simulink model "firefliesDemo"  (Simulink 7.4)
settings: Solver=ode3  StartTime=0.0  StopTime=200.0  FixedStep=0.5  RelTol=1e-3
values from neighbouring files (symbols this model uses):
  K = 0.1    [firefliesDemo.mat]
  N = 20    [firefliesDemo.mat]
  omega = 0.5    [firefliesDemo.mat]
  rho0 = 10    [firefliesDemo.mat]
  threshold = 4.71238898038    [firefliesDemo.mat]
  var = 10    [firefliesDemo.mat]
(part 1 of 2)
settings Model: Creator=chepeadan  LastModifiedBy=chepeadan
settings DataIOCC: SaveOutput=off  SaveState=on

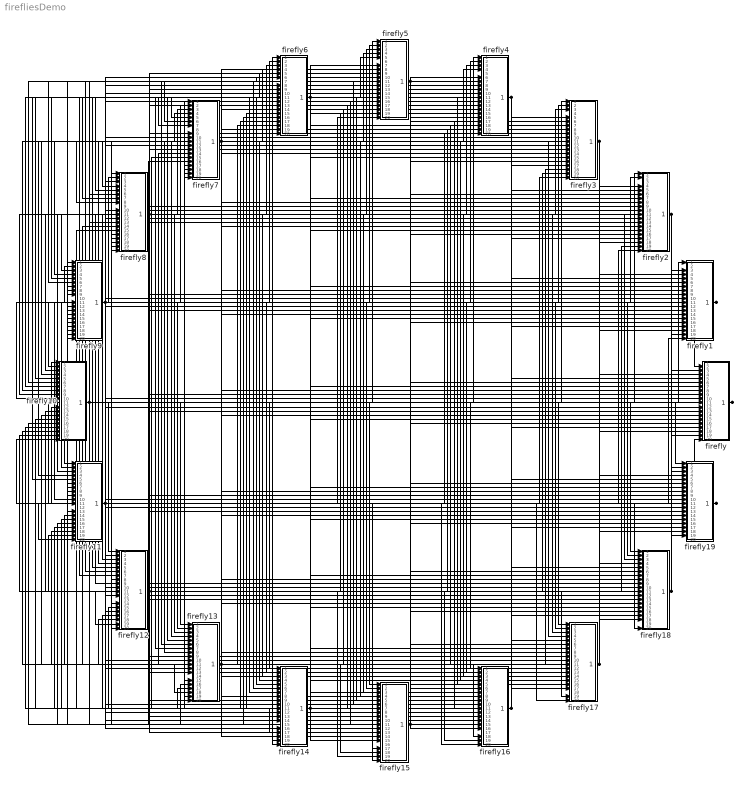
== system firefliesDemo ==
  firefly : Subsystem
  firefly1 : Subsystem
  firefly10 : Subsystem
  firefly11 : Subsystem
  firefly12 : Subsystem
  firefly13 : Subsystem
  firefly14 : Subsystem
  firefly15 : Subsystem
  firefly16 : Subsystem
  firefly17 : Subsystem
  firefly18 : Subsystem
  firefly19 : Subsystem
  firefly2 : Subsystem
  firefly3 : Subsystem
  firefly4 : Subsystem
  firefly5 : Subsystem
  firefly6 : Subsystem
  firefly7 : Subsystem
  firefly8 : Subsystem
  firefly9 : Subsystem
  wires:
  firefly/1(Out1) -> firefly1/1(In1), firefly2/1(In1), firefly3/1(In1), firefly4/1(In1), firefly5/1(In1), firefly6/1(In1), firefly7/1(In1), firefly8/1(In1), firefly9/1(In1), firefly10/1(In1), firefly11/1(In1), firefly12/1(In1), firefly13/1(In1), firefly14/1(In1), firefly15/1(In1), firefly16/1(In1), firefly17/1(In1), firefly18/1(In1), firefly19/1(In1)
  firefly1/1(Out1) -> firefly/2(In2), firefly2/2(In2), firefly3/2(In2), firefly4/2(In2), firefly5/2(In2), firefly6/2(In2), firefly7/2(In2), firefly8/2(In2), firefly9/2(In2), firefly10/2(In2), firefly11/2(In2), firefly12/2(In2), firefly13/2(In2), firefly14/2(In2), firefly15/2(In2), firefly16/2(In2), firefly17/2(In2), firefly18/2(In2), firefly19/2(In2)
  firefly2/1(Out1) -> firefly/3(In3), firefly1/3(In3), firefly3/3(In3), firefly4/3(In3), firefly5/3(In3), firefly6/3(In3), firefly7/3(In3), firefly8/3(In3), firefly9/3(In3), firefly10/3(In3), firefly11/3(In3), firefly12/3(In3), firefly13/3(In3), firefly14/3(In3), firefly15/3(In3), firefly16/3(In3), firefly17/3(In3), firefly18/3(In3), firefly19/3(In3)
  firefly3/1(Out1) -> firefly/4(In4), firefly1/4(In4), firefly2/4(In4), firefly4/4(In4), firefly5/4(In4), firefly6/4(In4), firefly7/4(In4), firefly8/4(In4), firefly9/4(In4), firefly10/4(In4), firefly11/4(In4), firefly12/4(In4), firefly13/4(In4), firefly14/4(In4), firefly15/4(In4), firefly16/4(In4), firefly17/4(In4), firefly18/4(In4), firefly19/4(In4)
  firefly4/1(Out1) -> firefly/5(In5), firefly1/5(In5), firefly2/5(In5), firefly3/5(In5), firefly5/5(In5), firefly6/5(In5), firefly7/5(In5), firefly8/5(In5), firefly9/5(In5), firefly10/5(In5), firefly11/5(In5), firefly12/5(In5), firefly13/5(In5), firefly14/5(In5), firefly15/5(In5), firefly16/5(In5), firefly17/5(In5), firefly18/5(In5), firefly19/5(In5)
  firefly5/1(Out1) -> firefly/6(In6), firefly1/6(In6), firefly2/6(In6), firefly3/6(In6), firefly4/6(In6), firefly6/6(In6), firefly7/6(In6), firefly8/6(In6), firefly9/6(In6), firefly10/6(In6), firefly11/6(In6), firefly12/6(In6), firefly13/6(In6), firefly14/6(In6), firefly15/6(In6), firefly16/6(In6), firefly17/6(In6), firefly18/6(In6), firefly19/6(In6)
  firefly6/1(Out1) -> firefly/7(In7), firefly1/7(In7), firefly2/7(In7), firefly3/7(In7), firefly4/7(In7), firefly5/7(In7), firefly7/7(In7), firefly8/7(In7), firefly9/7(In7), firefly10/7(In7), firefly11/7(In7), firefly12/7(In7), firefly13/7(In7), firefly14/7(In7), firefly15/7(In7), firefly16/7(In7), firefly17/7(In7), firefly18/7(In7), firefly19/7(In7)
  firefly7/1(Out1) -> firefly/8(In8), firefly1/8(In8), firefly2/8(In8), firefly3/8(In8), firefly4/8(In8), firefly5/8(In8), firefly6/8(In8), firefly8/8(In8), firefly9/8(In8), firefly10/8(In8), firefly11/8(In8), firefly12/8(In8), firefly13/8(In8), firefly14/8(In8), firefly15/8(In8), firefly16/8(In8), firefly17/8(In8), firefly18/8(In8), firefly19/8(In8)
  firefly8/1(Out1) -> firefly/9(In9), firefly1/9(In9), firefly2/9(In9), firefly3/9(In9), firefly4/9(In9), firefly5/9(In9), firefly6/9(In9), firefly7/9(In9), firefly9/9(In9), firefly10/9(In9), firefly11/9(In9), firefly12/9(In9), firefly13/9(In9), firefly14/9(In9), firefly15/9(In9), firefly16/9(In9), firefly17/9(In9), firefly18/9(In9), firefly19/9(In9)
  firefly9/1(Out1) -> firefly/10(In10), firefly1/10(In10), firefly2/10(In10), firefly3/10(In10), firefly4/10(In10), firefly5/10(In10), firefly6/10(In10), firefly7/10(In10), firefly8/10(In10), firefly10/10(In10), firefly11/10(In10), firefly12/10(In10), firefly13/10(In10), firefly14/10(In10), firefly15/10(In10), firefly16/10(In10), firefly17/10(In10), firefly18/10(In10), firefly19/10(In10)
  firefly10/1(Out1) -> firefly/11(In11), firefly1/11(In11), firefly2/11(In11), firefly3/11(In11), firefly4/11(In11), firefly5/11(In11), firefly6/11(In11), firefly7/11(In11), firefly8/11(In11), firefly9/11(In11), firefly11/11(In11), firefly12/11(In11), firefly13/11(In11), firefly14/11(In11), firefly15/11(In11), firefly16/11(In11), firefly17/11(In11), firefly18/11(In11), firefly19/11(In11)
  firefly11/1(Out1) -> firefly/12(In12), firefly1/12(In12), firefly2/12(In12), firefly3/12(In12), firefly4/12(In12), firefly5/12(In12), firefly6/12(In12), firefly7/12(In12), firefly8/12(In12), firefly9/12(In12), firefly10/12(In12), firefly12/12(In12), firefly13/12(In12), firefly14/12(In12), firefly15/12(In12), firefly16/12(In12), firefly17/12(In12), firefly18/12(In12), firefly19/12(In12)
  firefly12/1(Out1) -> firefly/13(In13), firefly1/13(In13), firefly2/13(In13), firefly3/13(In13), firefly4/13(In13), firefly5/13(In13), firefly6/13(In13), firefly7/13(In13), firefly8/13(In13), firefly9/13(In13), firefly10/13(In13), firefly11/13(In13), firefly13/13(In13), firefly14/13(In13), firefly15/13(In13), firefly16/13(In13), firefly17/13(In13), firefly18/13(In13), firefly19/13(In13)
  firefly13/1(Out1) -> firefly/14(In14), firefly1/14(In14), firefly2/14(In14), firefly3/14(In14), firefly4/14(In14), firefly5/14(In14), firefly6/14(In14), firefly7/14(In14), firefly8/14(In14), firefly9/14(In14), firefly10/14(In14), firefly11/14(In14), firefly12/14(In14), firefly14/14(In14), firefly15/14(In14), firefly16/14(In14), firefly17/14(In14), firefly18/14(In14), firefly19/14(In14)
  firefly14/1(Out1) -> firefly/15(In15), firefly1/15(In15), firefly2/15(In15), firefly3/15(In15), firefly4/15(In15), firefly5/15(In15), firefly6/15(In15), firefly7/15(In15), firefly8/15(In15), firefly9/15(In15), firefly10/15(In15), firefly11/15(In15), firefly12/15(In15), firefly13/15(In15), firefly15/15(In15), firefly16/15(In15), firefly17/15(In15), firefly18/15(In15), firefly19/15(In15)
  firefly15/1(Out1) -> firefly/16(In16), firefly1/16(In16), firefly2/16(In16), firefly3/16(In16), firefly4/16(In16), firefly5/16(In16), firefly6/16(In16), firefly7/16(In16), firefly8/16(In16), firefly9/16(In16), firefly10/16(In16), firefly11/16(In16), firefly12/16(In16), firefly13/16(In16), firefly14/16(In16), firefly16/16(In16), firefly17/16(In16), firefly18/16(In16), firefly19/16(In16)
  firefly16/1(Out1) -> firefly/17(In17), firefly1/17(In17), firefly2/17(In17), firefly3/17(In17), firefly4/17(In17), firefly5/17(In17), firefly6/17(In17), firefly7/17(In17), firefly8/17(In17), firefly9/17(In17), firefly10/17(In17), firefly11/17(In17), firefly12/17(In17), firefly13/17(In17), firefly14/17(In17), firefly15/17(In17), firefly17/17(In17), firefly18/17(In17), firefly19/17(In17)
  firefly17/1(Out1) -> firefly/18(In18), firefly1/18(In18), firefly2/18(In18), firefly3/18(In18), firefly4/18(In18), firefly5/18(In18), firefly6/18(In18), firefly7/18(In18), firefly8/18(In18), firefly9/18(In18), firefly10/18(In18), firefly11/18(In18), firefly12/18(In18), firefly13/18(In18), firefly14/18(In18), firefly15/18(In18), firefly16/18(In18), firefly18/18(In18), firefly19/18(In18)
  firefly18/1(Out1) -> firefly/19(In19), firefly1/19(In19), firefly2/19(In19), firefly3/19(In19), firefly4/19(In19), firefly5/19(In19), firefly6/19(In19), firefly7/19(In19), firefly8/19(In19), firefly9/19(In19), firefly10/19(In19), firefly11/19(In19), firefly12/19(In19), firefly13/19(In19), firefly14/19(In19), firefly15/19(In19), firefly16/19(In19), firefly17/19(In19), firefly19/19(In19)
  firefly19/1(Out1) -> firefly/20(In20), firefly1/20(In20), firefly2/20(In20), firefly3/20(In20), firefly4/20(In20), firefly5/20(In20), firefly6/20(In20), firefly7/20(In20), firefly8/20(In20), firefly9/20(In20), firefly10/20(In20), firefly11/20(In20), firefly12/20(In20), firefly13/20(In20), firefly14/20(In20), firefly15/20(In20), firefly16/20(In20), firefly17/20(In20), firefly18/20(In20)

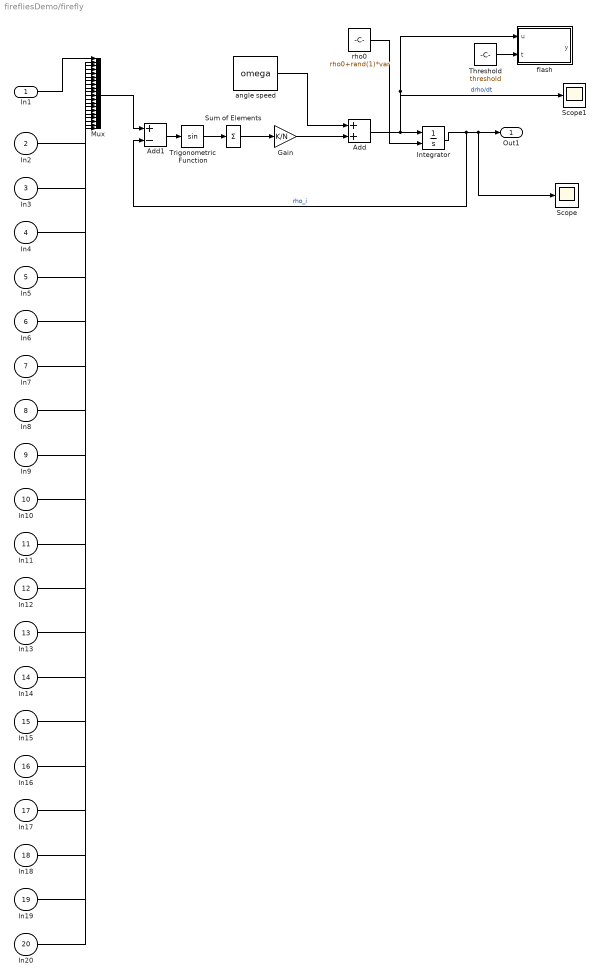
== system firefliesDemo/firefly ==
  In1 : Inport  OutDataType=fixdt(1, 16)  OutScaling=2^0
  In2 : Inport  Port=2
  In3 : Inport  Port=3
  In4 : Inport  Port=4
  In5 : Inport  Port=5
  In6 : Inport  Port=6
  In7 : Inport  Port=7
  In8 : Inport  Port=8
  In9 : Inport  Port=9
  In10 : Inport  Port=10
  In11 : Inport  Port=11
  In12 : Inport  Port=12
  In13 : Inport  Port=13
  In14 : Inport  Port=14
  In15 : Inport  Port=15
  In16 : Inport  Port=16
  In17 : Inport  Port=17
  In18 : Inport  Port=18
  In19 : Inport  Port=19
  In20 : Inport  Port=20
  Add : Sum  OutDataType=fixdt(1, 16)  OutScaling=2^-10
  Add1 : Sum  Inputs=+-  OutDataType=fixdt(1, 16)  OutScaling=2^-10
  Gain : Gain  Gain=K/N  ParameterDataType=fixdt(1, 16)  ParameterScaling=2^0  OutDataType=fixdt(1, 16)  OutScaling=2^0
  Integrator : Integrator  InitialConditionSource=external
  Mux : Mux  Inputs=20
  Scope : Scope
  Scope1 : Scope
  Sum of Elements : Sum  Inputs=+  OutDataType=fixdt(1, 16)  OutScaling=2^-10
  Threshold : Constant  Value=threshold  OutDataType=fixdt(1, 16)  OutScaling=2^0
  Trigonometric Function : Trigonometry
  angle speed : Constant  Value=omega  OutDataType=fixdt(1, 16)  OutScaling=2^0
  flash : Stateflow chart
  rho0 : Constant  Value=rho0+rand(1)*var  OutDataType=fixdt(1, 16)  OutScaling=2^0
  Out1 : Outport  OutDataType=fixdt(1, 16)  OutScaling=2^0
  wires:
  In20/1 -> Mux/20
  In19/1 -> Mux/19
  In18/1 -> Mux/18
  In17/1 -> Mux/17
  In16/1 -> Mux/16
  In15/1 -> Mux/15
  In14/1 -> Mux/14
  In13/1 -> Mux/13
  In12/1 -> Mux/12
  In11/1 -> Mux/11
  In10/1 -> Mux/10
  In9/1 -> Mux/9
  In8/1 -> Mux/8
  In7/1 -> Mux/7
  In6/1 -> Mux/6
  In5/1 -> Mux/5
  In4/1 -> Mux/4
  In3/1 -> Mux/3
  In2/1 -> Mux/2
  rho0/1 -> Integrator/2
  Threshold/1 -> flash/2(t)
  Sum of Elements/1 -> Gain/1
  Trigonometric Function/1 -> Sum of Elements/1
  Add/1 -> Scope1/1, flash/1(u), Integrator/1  "drho/dt"
  Gain/1 -> Add/2
  angle speed/1 -> Add/1
  Add1/1 -> Trigonometric Function/1
  Integrator/1 -> Scope/1, Out1/1, Add1/2  "rho_i"
  Mux/1 -> Add1/1
  In1/1 -> Mux/1

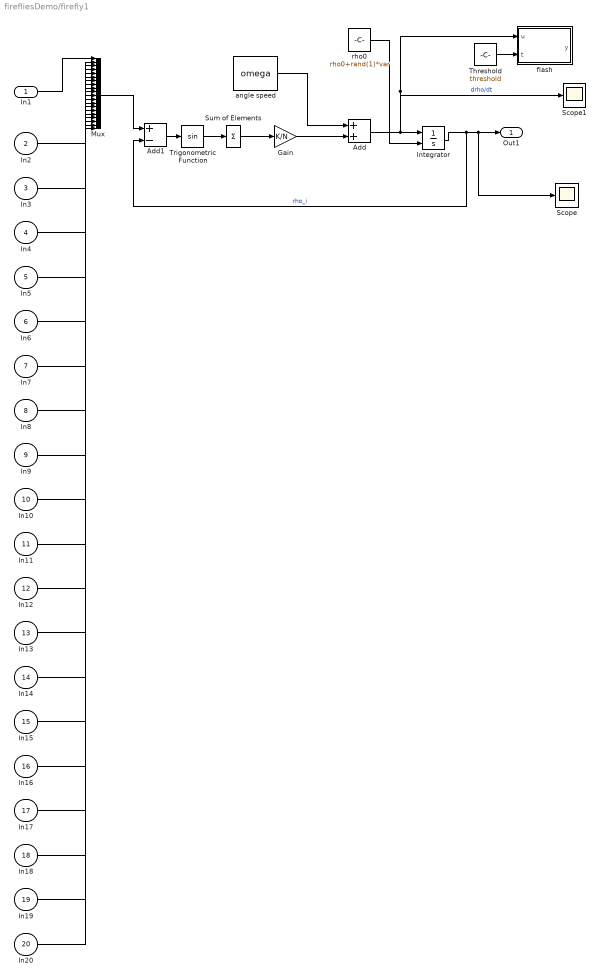
== system firefliesDemo/firefly1 ==
  In1 : Inport  OutDataType=fixdt(1, 16)  OutScaling=2^0
  In2 : Inport  Port=2
  In3 : Inport  Port=3
  In4 : Inport  Port=4
  In5 : Inport  Port=5
  In6 : Inport  Port=6
  In7 : Inport  Port=7
  In8 : Inport  Port=8
  In9 : Inport  Port=9
  In10 : Inport  Port=10
  In11 : Inport  Port=11
  In12 : Inport  Port=12
  In13 : Inport  Port=13
  In14 : Inport  Port=14
  In15 : Inport  Port=15
  In16 : Inport  Port=16
  In17 : Inport  Port=17
  In18 : Inport  Port=18
  In19 : Inport  Port=19
  In20 : Inport  Port=20
  Add : Sum  OutDataType=fixdt(1, 16)  OutScaling=2^-10
  Add1 : Sum  Inputs=+-  OutDataType=fixdt(1, 16)  OutScaling=2^-10
  Gain : Gain  Gain=K/N  ParameterDataType=fixdt(1, 16)  ParameterScaling=2^0  OutDataType=fixdt(1, 16)  OutScaling=2^0
  Integrator : Integrator  InitialConditionSource=external
  Mux : Mux  Inputs=20
  Scope : Scope
  Scope1 : Scope
  Sum of Elements : Sum  Inputs=+  OutDataType=fixdt(1, 16)  OutScaling=2^-10
  Threshold : Constant  Value=threshold  OutDataType=fixdt(1, 16)  OutScaling=2^0
  Trigonometric Function : Trigonometry
  angle speed : Constant  Value=omega  OutDataType=fixdt(1, 16)  OutScaling=2^0
  flash : Stateflow chart
  rho0 : Constant  Value=rho0+rand(1)*var  OutDataType=fixdt(1, 16)  OutScaling=2^0
  Out1 : Outport  OutDataType=fixdt(1, 16)  OutScaling=2^0
  wires:
  In20/1 -> Mux/20
  In19/1 -> Mux/19
  In18/1 -> Mux/18
  In17/1 -> Mux/17
  In16/1 -> Mux/16
  In15/1 -> Mux/15
  In14/1 -> Mux/14
  In13/1 -> Mux/13
  In12/1 -> Mux/12
  In11/1 -> Mux/11
  In10/1 -> Mux/10
  In9/1 -> Mux/9
  In8/1 -> Mux/8
  In7/1 -> Mux/7
  In6/1 -> Mux/6
  In5/1 -> Mux/5
  In4/1 -> Mux/4
  In3/1 -> Mux/3
  In2/1 -> Mux/2
  rho0/1 -> Integrator/2
  Threshold/1 -> flash/2(t)
  Sum of Elements/1 -> Gain/1
  Trigonometric Function/1 -> Sum of Elements/1
  Add/1 -> Scope1/1, flash/1(u), Integrator/1  "drho/dt"
  Gain/1 -> Add/2
  angle speed/1 -> Add/1
  Add1/1 -> Trigonometric Function/1
  Integrator/1 -> Scope/1, Out1/1, Add1/2  "rho_i"
  Mux/1 -> Add1/1
  In1/1 -> Mux/1

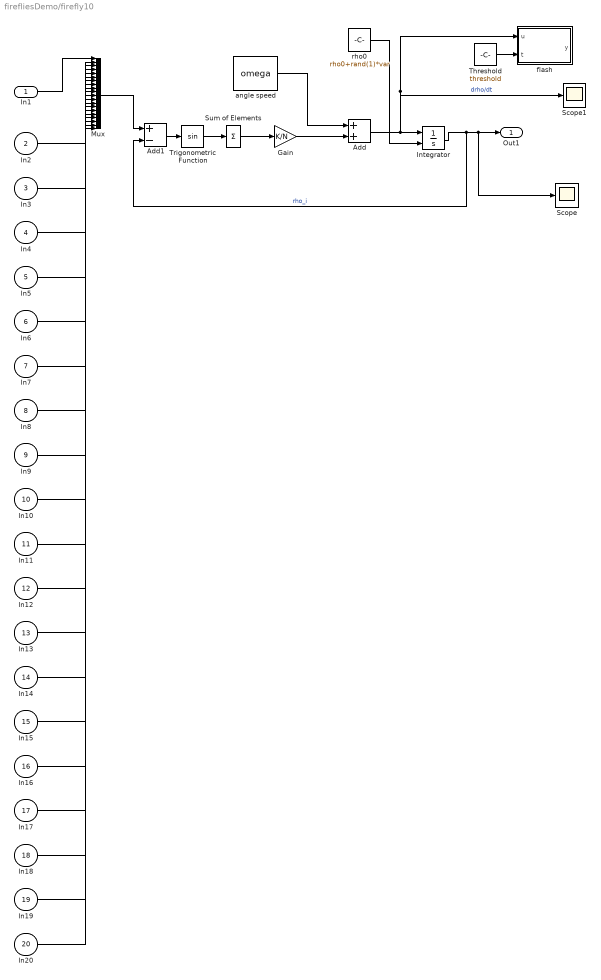
== system firefliesDemo/firefly10 ==
  In1 : Inport  OutDataType=fixdt(1, 16)  OutScaling=2^0
  In2 : Inport  Port=2
  In3 : Inport  Port=3
  In4 : Inport  Port=4
  In5 : Inport  Port=5
  In6 : Inport  Port=6
  In7 : Inport  Port=7
  In8 : Inport  Port=8
  In9 : Inport  Port=9
  In10 : Inport  Port=10
  In11 : Inport  Port=11
  In12 : Inport  Port=12
  In13 : Inport  Port=13
  In14 : Inport  Port=14
  In15 : Inport  Port=15
  In16 : Inport  Port=16
  In17 : Inport  Port=17
  In18 : Inport  Port=18
  In19 : Inport  Port=19
  In20 : Inport  Port=20
  Add : Sum  OutDataType=fixdt(1, 16)  OutScaling=2^-10
  Add1 : Sum  Inputs=+-  OutDataType=fixdt(1, 16)  OutScaling=2^-10
  Gain : Gain  Gain=K/N  ParameterDataType=fixdt(1, 16)  ParameterScaling=2^0  OutDataType=fixdt(1, 16)  OutScaling=2^0
  Integrator : Integrator  InitialConditionSource=external
  Mux : Mux  Inputs=20
  Scope : Scope
  Scope1 : Scope
  Sum of Elements : Sum  Inputs=+  OutDataType=fixdt(1, 16)  OutScaling=2^-10
  Threshold : Constant  Value=threshold  OutDataType=fixdt(1, 16)  OutScaling=2^0
  Trigonometric Function : Trigonometry
  angle speed : Constant  Value=omega  OutDataType=fixdt(1, 16)  OutScaling=2^0
  flash : Stateflow chart
  rho0 : Constant  Value=rho0+rand(1)*var  OutDataType=fixdt(1, 16)  OutScaling=2^0
  Out1 : Outport  OutDataType=fixdt(1, 16)  OutScaling=2^0
  wires:
  In20/1 -> Mux/20
  In19/1 -> Mux/19
  In18/1 -> Mux/18
  In17/1 -> Mux/17
  In16/1 -> Mux/16
  In15/1 -> Mux/15
  In14/1 -> Mux/14
  In13/1 -> Mux/13
  In12/1 -> Mux/12
  In11/1 -> Mux/11
  In10/1 -> Mux/10
  In9/1 -> Mux/9
  In8/1 -> Mux/8
  In7/1 -> Mux/7
  In6/1 -> Mux/6
  In5/1 -> Mux/5
  In4/1 -> Mux/4
  In3/1 -> Mux/3
  In2/1 -> Mux/2
  rho0/1 -> Integrator/2
  Threshold/1 -> flash/2(t)
  Sum of Elements/1 -> Gain/1
  Trigonometric Function/1 -> Sum of Elements/1
  Add/1 -> Scope1/1, flash/1(u), Integrator/1  "drho/dt"
  Gain/1 -> Add/2
  angle speed/1 -> Add/1
  Add1/1 -> Trigonometric Function/1
  Integrator/1 -> Scope/1, Out1/1, Add1/2  "rho_i"
  Mux/1 -> Add1/1
  In1/1 -> Mux/1

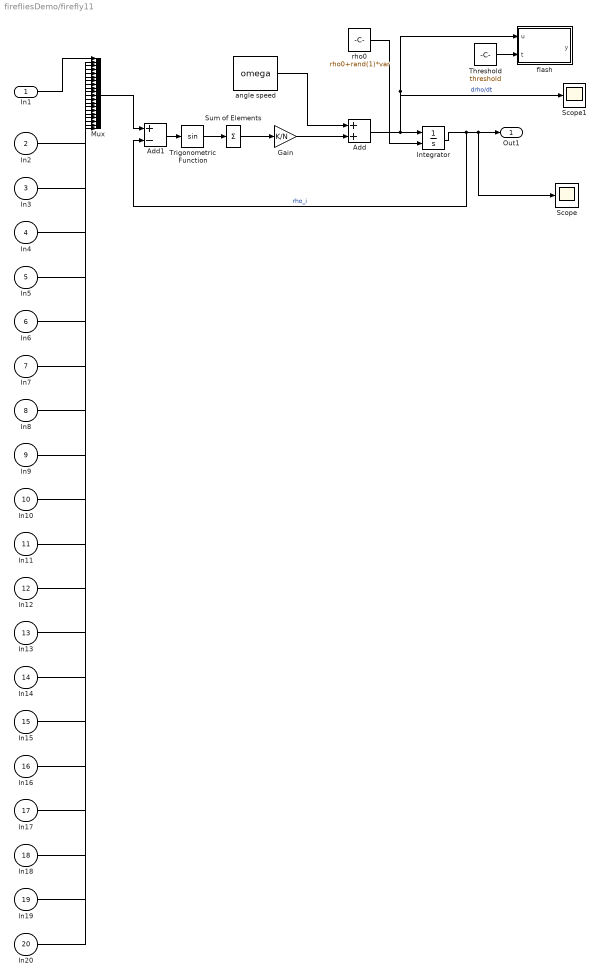
== system firefliesDemo/firefly11 ==
  In1 : Inport  OutDataType=fixdt(1, 16)  OutScaling=2^0
  In2 : Inport  Port=2
  In3 : Inport  Port=3
  In4 : Inport  Port=4
  In5 : Inport  Port=5
  In6 : Inport  Port=6
  In7 : Inport  Port=7
  In8 : Inport  Port=8
  In9 : Inport  Port=9
  In10 : Inport  Port=10
  In11 : Inport  Port=11
  In12 : Inport  Port=12
  In13 : Inport  Port=13
  In14 : Inport  Port=14
  In15 : Inport  Port=15
  In16 : Inport  Port=16
  In17 : Inport  Port=17
  In18 : Inport  Port=18
  In19 : Inport  Port=19
  In20 : Inport  Port=20
  Add : Sum  OutDataType=fixdt(1, 16)  OutScaling=2^-10
  Add1 : Sum  Inputs=+-  OutDataType=fixdt(1, 16)  OutScaling=2^-10
  Gain : Gain  Gain=K/N  ParameterDataType=fixdt(1, 16)  ParameterScaling=2^0  OutDataType=fixdt(1, 16)  OutScaling=2^0
  Integrator : Integrator  InitialConditionSource=external
  Mux : Mux  Inputs=20
  Scope : Scope
  Scope1 : Scope
  Sum of Elements : Sum  Inputs=+  OutDataType=fixdt(1, 16)  OutScaling=2^-10
  Threshold : Constant  Value=threshold  OutDataType=fixdt(1, 16)  OutScaling=2^0
  Trigonometric Function : Trigonometry
  angle speed : Constant  Value=omega  OutDataType=fixdt(1, 16)  OutScaling=2^0
  flash : Stateflow chart
  rho0 : Constant  Value=rho0+rand(1)*var  OutDataType=fixdt(1, 16)  OutScaling=2^0
  Out1 : Outport  OutDataType=fixdt(1, 16)  OutScaling=2^0
  wires:
  In20/1 -> Mux/20
  In19/1 -> Mux/19
  In18/1 -> Mux/18
  In17/1 -> Mux/17
  In16/1 -> Mux/16
  In15/1 -> Mux/15
  In14/1 -> Mux/14
  In13/1 -> Mux/13
  In12/1 -> Mux/12
  In11/1 -> Mux/11
  In10/1 -> Mux/10
  In9/1 -> Mux/9
  In8/1 -> Mux/8
  In7/1 -> Mux/7
  In6/1 -> Mux/6
  In5/1 -> Mux/5
  In4/1 -> Mux/4
  In3/1 -> Mux/3
  In2/1 -> Mux/2
  rho0/1 -> Integrator/2
  Threshold/1 -> flash/2(t)
  Sum of Elements/1 -> Gain/1
  Trigonometric Function/1 -> Sum of Elements/1
  Add/1 -> Scope1/1, flash/1(u), Integrator/1  "drho/dt"
  Gain/1 -> Add/2
  angle speed/1 -> Add/1
  Add1/1 -> Trigonometric Function/1
  Integrator/1 -> Scope/1, Out1/1, Add1/2  "rho_i"
  Mux/1 -> Add1/1
  In1/1 -> Mux/1

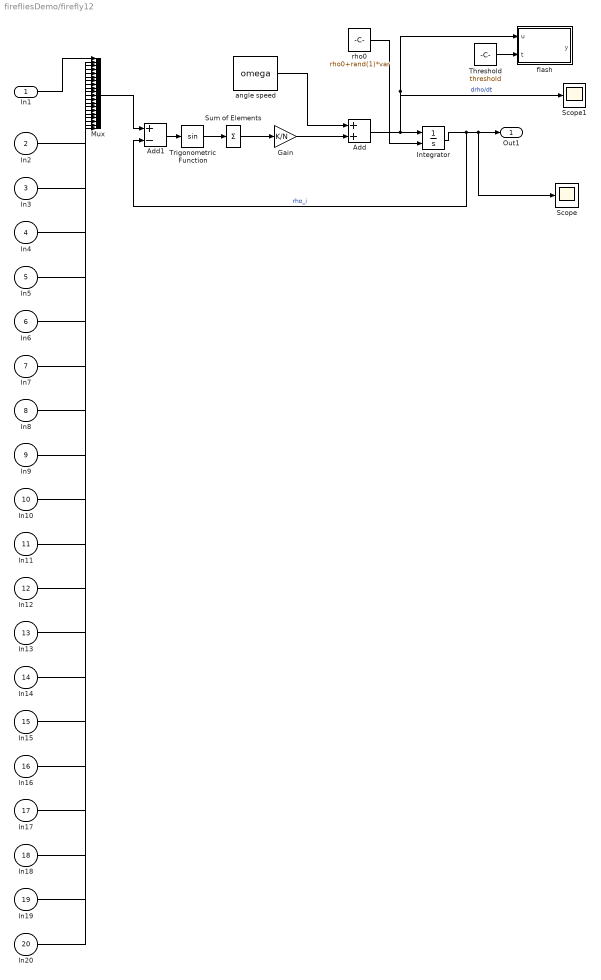
== system firefliesDemo/firefly12 ==
  In1 : Inport  OutDataType=fixdt(1, 16)  OutScaling=2^0
  In2 : Inport  Port=2
  In3 : Inport  Port=3
  In4 : Inport  Port=4
  In5 : Inport  Port=5
  In6 : Inport  Port=6
  In7 : Inport  Port=7
  In8 : Inport  Port=8
  In9 : Inport  Port=9
  In10 : Inport  Port=10
  In11 : Inport  Port=11
  In12 : Inport  Port=12
  In13 : Inport  Port=13
  In14 : Inport  Port=14
  In15 : Inport  Port=15
  In16 : Inport  Port=16
  In17 : Inport  Port=17
  In18 : Inport  Port=18
  In19 : Inport  Port=19
  In20 : Inport  Port=20
  Add : Sum  OutDataType=fixdt(1, 16)  OutScaling=2^-10
  Add1 : Sum  Inputs=+-  OutDataType=fixdt(1, 16)  OutScaling=2^-10
  Gain : Gain  Gain=K/N  ParameterDataType=fixdt(1, 16)  ParameterScaling=2^0  OutDataType=fixdt(1, 16)  OutScaling=2^0
  Integrator : Integrator  InitialConditionSource=external
  Mux : Mux  Inputs=20
  Scope : Scope
  Scope1 : Scope
  Sum of Elements : Sum  Inputs=+  OutDataType=fixdt(1, 16)  OutScaling=2^-10
  Threshold : Constant  Value=threshold  OutDataType=fixdt(1, 16)  OutScaling=2^0
  Trigonometric Function : Trigonometry
  angle speed : Constant  Value=omega  OutDataType=fixdt(1, 16)  OutScaling=2^0
  flash : Stateflow chart
  rho0 : Constant  Value=rho0+rand(1)*var  OutDataType=fixdt(1, 16)  OutScaling=2^0
  Out1 : Outport  OutDataType=fixdt(1, 16)  OutScaling=2^0
  wires:
  In20/1 -> Mux/20
  In19/1 -> Mux/19
  In18/1 -> Mux/18
  In17/1 -> Mux/17
  In16/1 -> Mux/16
  In15/1 -> Mux/15
  In14/1 -> Mux/14
  In13/1 -> Mux/13
  In12/1 -> Mux/12
  In11/1 -> Mux/11
  In10/1 -> Mux/10
  In9/1 -> Mux/9
  In8/1 -> Mux/8
  In7/1 -> Mux/7
  In6/1 -> Mux/6
  In5/1 -> Mux/5
  In4/1 -> Mux/4
  In3/1 -> Mux/3
  In2/1 -> Mux/2
  rho0/1 -> Integrator/2
  Threshold/1 -> flash/2(t)
  Sum of Elements/1 -> Gain/1
  Trigonometric Function/1 -> Sum of Elements/1
  Add/1 -> Scope1/1, flash/1(u), Integrator/1  "drho/dt"
  Gain/1 -> Add/2
  angle speed/1 -> Add/1
  Add1/1 -> Trigonometric Function/1
  Integrator/1 -> Scope/1, Out1/1, Add1/2  "rho_i"
  Mux/1 -> Add1/1
  In1/1 -> Mux/1

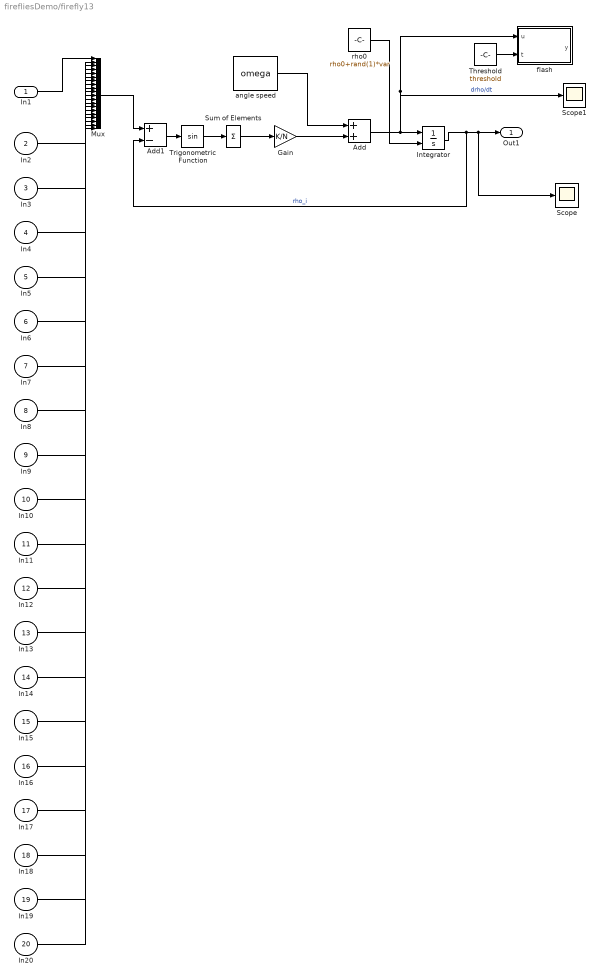
== system firefliesDemo/firefly13 ==
  In1 : Inport  OutDataType=fixdt(1, 16)  OutScaling=2^0
  In2 : Inport  Port=2
  In3 : Inport  Port=3
  In4 : Inport  Port=4
  In5 : Inport  Port=5
  In6 : Inport  Port=6
  In7 : Inport  Port=7
  In8 : Inport  Port=8
  In9 : Inport  Port=9
  In10 : Inport  Port=10
  In11 : Inport  Port=11
  In12 : Inport  Port=12
  In13 : Inport  Port=13
  In14 : Inport  Port=14
  In15 : Inport  Port=15
  In16 : Inport  Port=16
  In17 : Inport  Port=17
  In18 : Inport  Port=18
  In19 : Inport  Port=19
  In20 : Inport  Port=20
  Add : Sum  OutDataType=fixdt(1, 16)  OutScaling=2^-10
  Add1 : Sum  Inputs=+-  OutDataType=fixdt(1, 16)  OutScaling=2^-10
  Gain : Gain  Gain=K/N  ParameterDataType=fixdt(1, 16)  ParameterScaling=2^0  OutDataType=fixdt(1, 16)  OutScaling=2^0
  Integrator : Integrator  InitialConditionSource=external
  Mux : Mux  Inputs=20
  Scope : Scope
  Scope1 : Scope
  Sum of Elements : Sum  Inputs=+  OutDataType=fixdt(1, 16)  OutScaling=2^-10
  Threshold : Constant  Value=threshold  OutDataType=fixdt(1, 16)  OutScaling=2^0
  Trigonometric Function : Trigonometry
  angle speed : Constant  Value=omega  OutDataType=fixdt(1, 16)  OutScaling=2^0
  flash : Stateflow chart
  rho0 : Constant  Value=rho0+rand(1)*var  OutDataType=fixdt(1, 16)  OutScaling=2^0
  Out1 : Outport  OutDataType=fixdt(1, 16)  OutScaling=2^0
  wires:
  In20/1 -> Mux/20
  In19/1 -> Mux/19
  In18/1 -> Mux/18
  In17/1 -> Mux/17
  In16/1 -> Mux/16
  In15/1 -> Mux/15
  In14/1 -> Mux/14
  In13/1 -> Mux/13
  In12/1 -> Mux/12
  In11/1 -> Mux/11
  In10/1 -> Mux/10
  In9/1 -> Mux/9
  In8/1 -> Mux/8
  In7/1 -> Mux/7
  In6/1 -> Mux/6
  In5/1 -> Mux/5
  In4/1 -> Mux/4
  In3/1 -> Mux/3
  In2/1 -> Mux/2
  rho0/1 -> Integrator/2
  Threshold/1 -> flash/2(t)
  Sum of Elements/1 -> Gain/1
  Trigonometric Function/1 -> Sum of Elements/1
  Add/1 -> Scope1/1, flash/1(u), Integrator/1  "drho/dt"
  Gain/1 -> Add/2
  angle speed/1 -> Add/1
  Add1/1 -> Trigonometric Function/1
  Integrator/1 -> Scope/1, Out1/1, Add1/2  "rho_i"
  Mux/1 -> Add1/1
  In1/1 -> Mux/1

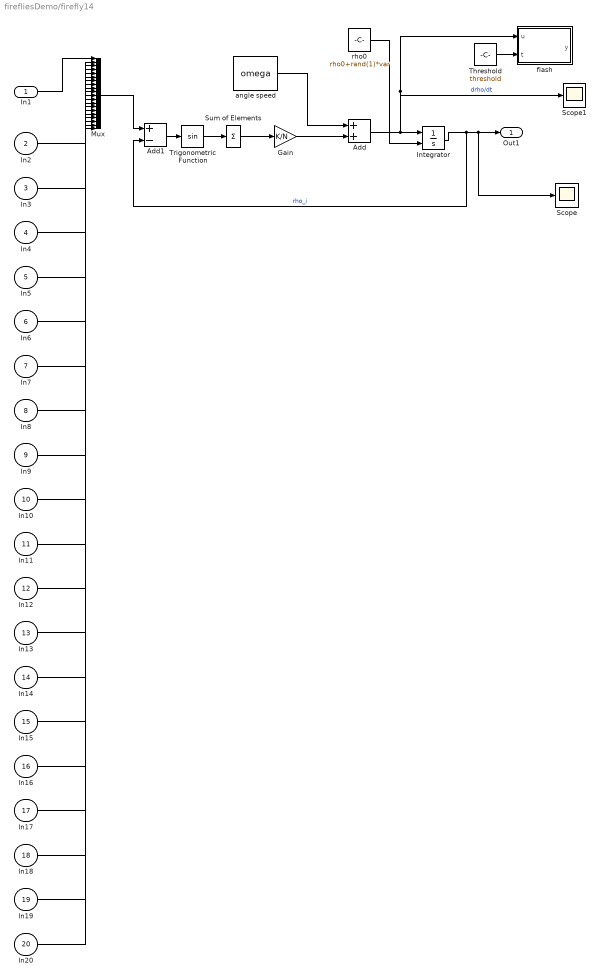
== system firefliesDemo/firefly14 ==
  In1 : Inport  OutDataType=fixdt(1, 16)  OutScaling=2^0
  In2 : Inport  Port=2
  In3 : Inport  Port=3
  In4 : Inport  Port=4
  In5 : Inport  Port=5
  In6 : Inport  Port=6
  In7 : Inport  Port=7
  In8 : Inport  Port=8
  In9 : Inport  Port=9
  In10 : Inport  Port=10
  In11 : Inport  Port=11
  In12 : Inport  Port=12
  In13 : Inport  Port=13
  In14 : Inport  Port=14
  In15 : Inport  Port=15
  In16 : Inport  Port=16
  In17 : Inport  Port=17
  In18 : Inport  Port=18
  In19 : Inport  Port=19
  In20 : Inport  Port=20
  Add : Sum  OutDataType=fixdt(1, 16)  OutScaling=2^-10
  Add1 : Sum  Inputs=+-  OutDataType=fixdt(1, 16)  OutScaling=2^-10
  Gain : Gain  Gain=K/N  ParameterDataType=fixdt(1, 16)  ParameterScaling=2^0  OutDataType=fixdt(1, 16)  OutScaling=2^0
  Integrator : Integrator  InitialConditionSource=external
  Mux : Mux  Inputs=20
  Scope : Scope
  Scope1 : Scope
  Sum of Elements : Sum  Inputs=+  OutDataType=fixdt(1, 16)  OutScaling=2^-10
  Threshold : Constant  Value=threshold  OutDataType=fixdt(1, 16)  OutScaling=2^0
  Trigonometric Function : Trigonometry
  angle speed : Constant  Value=omega  OutDataType=fixdt(1, 16)  OutScaling=2^0
  flash : Stateflow chart
  rho0 : Constant  Value=rho0+rand(1)*var  OutDataType=fixdt(1, 16)  OutScaling=2^0
  Out1 : Outport  OutDataType=fixdt(1, 16)  OutScaling=2^0
  wires:
  In20/1 -> Mux/20
  In19/1 -> Mux/19
  In18/1 -> Mux/18
  In17/1 -> Mux/17
  In16/1 -> Mux/16
  In15/1 -> Mux/15
  In14/1 -> Mux/14
  In13/1 -> Mux/13
  In12/1 -> Mux/12
  In11/1 -> Mux/11
  In10/1 -> Mux/10
  In9/1 -> Mux/9
  In8/1 -> Mux/8
  In7/1 -> Mux/7
  In6/1 -> Mux/6
  In5/1 -> Mux/5
  In4/1 -> Mux/4
  In3/1 -> Mux/3
  In2/1 -> Mux/2
  rho0/1 -> Integrator/2
  Threshold/1 -> flash/2(t)
  Sum of Elements/1 -> Gain/1
  Trigonometric Function/1 -> Sum of Elements/1
  Add/1 -> Scope1/1, flash/1(u), Integrator/1  "drho/dt"
  Gain/1 -> Add/2
  angle speed/1 -> Add/1
  Add1/1 -> Trigonometric Function/1
  Integrator/1 -> Scope/1, Out1/1, Add1/2  "rho_i"
  Mux/1 -> Add1/1
  In1/1 -> Mux/1

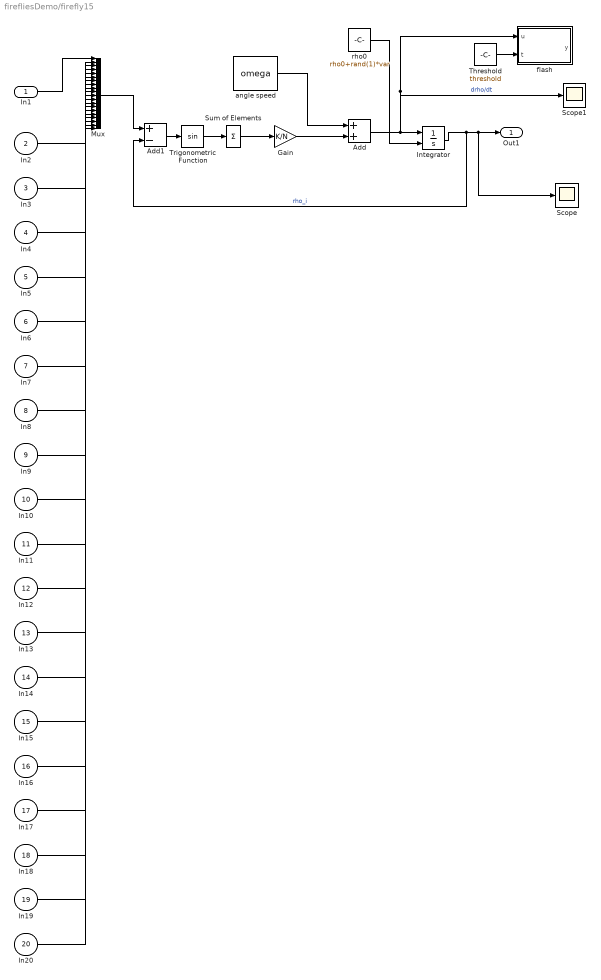
== system firefliesDemo/firefly15 ==
  In1 : Inport  OutDataType=fixdt(1, 16)  OutScaling=2^0
  In2 : Inport  Port=2
  In3 : Inport  Port=3
  In4 : Inport  Port=4
  In5 : Inport  Port=5
  In6 : Inport  Port=6
  In7 : Inport  Port=7
  In8 : Inport  Port=8
  In9 : Inport  Port=9
  In10 : Inport  Port=10
  In11 : Inport  Port=11
  In12 : Inport  Port=12
  In13 : Inport  Port=13
  In14 : Inport  Port=14
  In15 : Inport  Port=15
  In16 : Inport  Port=16
  In17 : Inport  Port=17
  In18 : Inport  Port=18
  In19 : Inport  Port=19
  In20 : Inport  Port=20
  Add : Sum  OutDataType=fixdt(1, 16)  OutScaling=2^-10
  Add1 : Sum  Inputs=+-  OutDataType=fixdt(1, 16)  OutScaling=2^-10
  Gain : Gain  Gain=K/N  ParameterDataType=fixdt(1, 16)  ParameterScaling=2^0  OutDataType=fixdt(1, 16)  OutScaling=2^0
  Integrator : Integrator  InitialConditionSource=external
  Mux : Mux  Inputs=20
  Scope : Scope
  Scope1 : Scope
  Sum of Elements : Sum  Inputs=+  OutDataType=fixdt(1, 16)  OutScaling=2^-10
  Threshold : Constant  Value=threshold  OutDataType=fixdt(1, 16)  OutScaling=2^0
  Trigonometric Function : Trigonometry
  angle speed : Constant  Value=omega  OutDataType=fixdt(1, 16)  OutScaling=2^0
  flash : Stateflow chart
  rho0 : Constant  Value=rho0+rand(1)*var  OutDataType=fixdt(1, 16)  OutScaling=2^0
  Out1 : Outport  OutDataType=fixdt(1, 16)  OutScaling=2^0
  wires:
  In20/1 -> Mux/20
  In19/1 -> Mux/19
  In18/1 -> Mux/18
  In17/1 -> Mux/17
  In16/1 -> Mux/16
  In15/1 -> Mux/15
  In14/1 -> Mux/14
  In13/1 -> Mux/13
  In12/1 -> Mux/12
  In11/1 -> Mux/11
  In10/1 -> Mux/10
  In9/1 -> Mux/9
  In8/1 -> Mux/8
  In7/1 -> Mux/7
  In6/1 -> Mux/6
  In5/1 -> Mux/5
  In4/1 -> Mux/4
  In3/1 -> Mux/3
  In2/1 -> Mux/2
  rho0/1 -> Integrator/2
  Threshold/1 -> flash/2(t)
  Sum of Elements/1 -> Gain/1
  Trigonometric Function/1 -> Sum of Elements/1
  Add/1 -> Scope1/1, flash/1(u), Integrator/1  "drho/dt"
  Gain/1 -> Add/2
  angle speed/1 -> Add/1
  Add1/1 -> Trigonometric Function/1
  Integrator/1 -> Scope/1, Out1/1, Add1/2  "rho_i"
  Mux/1 -> Add1/1
  In1/1 -> Mux/1

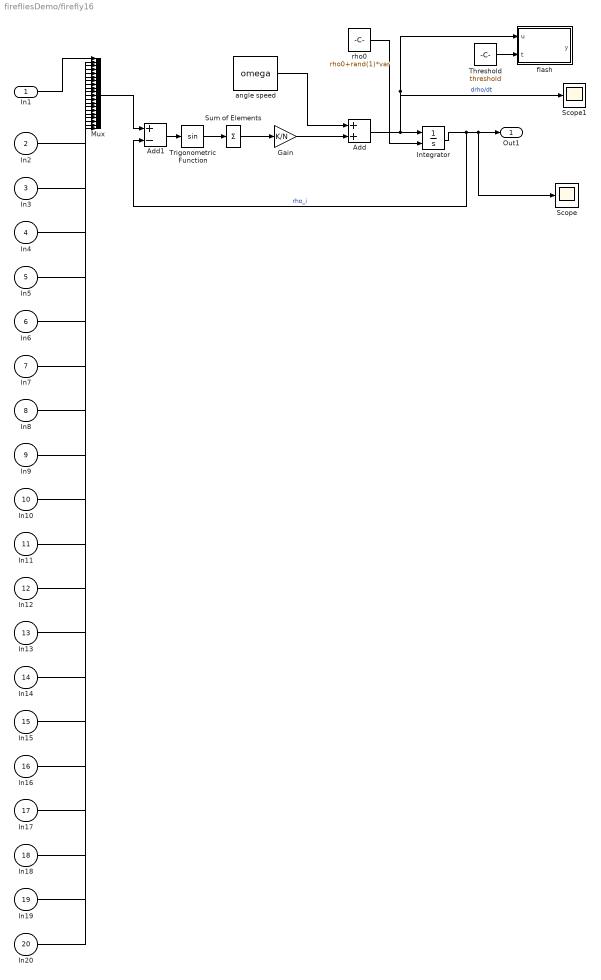
== system firefliesDemo/firefly16 ==
  In1 : Inport  OutDataType=fixdt(1, 16)  OutScaling=2^0
  In2 : Inport  Port=2
  In3 : Inport  Port=3
  In4 : Inport  Port=4
  In5 : Inport  Port=5
  In6 : Inport  Port=6
  In7 : Inport  Port=7
  In8 : Inport  Port=8
  In9 : Inport  Port=9
  In10 : Inport  Port=10
  In11 : Inport  Port=11
  In12 : Inport  Port=12
  In13 : Inport  Port=13
  In14 : Inport  Port=14
  In15 : Inport  Port=15
  In16 : Inport  Port=16
  In17 : Inport  Port=17
  In18 : Inport  Port=18
  In19 : Inport  Port=19
  In20 : Inport  Port=20
  Add : Sum  OutDataType=fixdt(1, 16)  OutScaling=2^-10
  Add1 : Sum  Inputs=+-  OutDataType=fixdt(1, 16)  OutScaling=2^-10
  Gain : Gain  Gain=K/N  ParameterDataType=fixdt(1, 16)  ParameterScaling=2^0  OutDataType=fixdt(1, 16)  OutScaling=2^0
  Integrator : Integrator  InitialConditionSource=external
  Mux : Mux  Inputs=20
  Scope : Scope
  Scope1 : Scope
  Sum of Elements : Sum  Inputs=+  OutDataType=fixdt(1, 16)  OutScaling=2^-10
  Threshold : Constant  Value=threshold  OutDataType=fixdt(1, 16)  OutScaling=2^0
  Trigonometric Function : Trigonometry
  angle speed : Constant  Value=omega  OutDataType=fixdt(1, 16)  OutScaling=2^0
  flash : Stateflow chart
  rho0 : Constant  Value=rho0+rand(1)*var  OutDataType=fixdt(1, 16)  OutScaling=2^0
  Out1 : Outport  OutDataType=fixdt(1, 16)  OutScaling=2^0
  wires:
  In20/1 -> Mux/20
  In19/1 -> Mux/19
  In18/1 -> Mux/18
  In17/1 -> Mux/17
  In16/1 -> Mux/16
  In15/1 -> Mux/15
  In14/1 -> Mux/14
  In13/1 -> Mux/13
  In12/1 -> Mux/12
  In11/1 -> Mux/11
  In10/1 -> Mux/10
  In9/1 -> Mux/9
  In8/1 -> Mux/8
  In7/1 -> Mux/7
  In6/1 -> Mux/6
  In5/1 -> Mux/5
  In4/1 -> Mux/4
  In3/1 -> Mux/3
  In2/1 -> Mux/2
  rho0/1 -> Integrator/2
  Threshold/1 -> flash/2(t)
  Sum of Elements/1 -> Gain/1
  Trigonometric Function/1 -> Sum of Elements/1
  Add/1 -> Scope1/1, flash/1(u), Integrator/1  "drho/dt"
  Gain/1 -> Add/2
  angle speed/1 -> Add/1
  Add1/1 -> Trigonometric Function/1
  Integrator/1 -> Scope/1, Out1/1, Add1/2  "rho_i"
  Mux/1 -> Add1/1
  In1/1 -> Mux/1

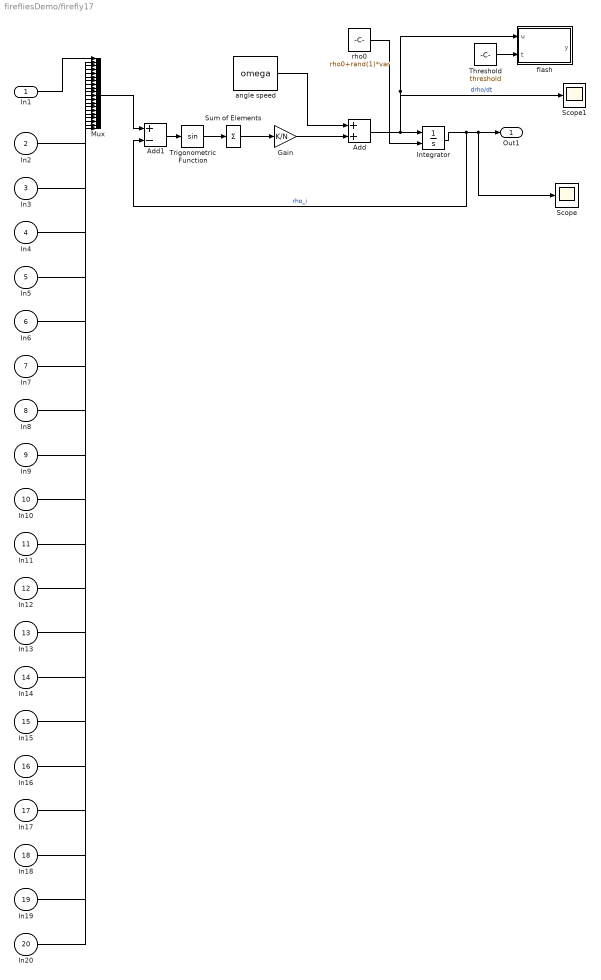
== system firefliesDemo/firefly17 ==
  In1 : Inport  OutDataType=fixdt(1, 16)  OutScaling=2^0
  In2 : Inport  Port=2
  In3 : Inport  Port=3
  In4 : Inport  Port=4
  In5 : Inport  Port=5
  In6 : Inport  Port=6
  In7 : Inport  Port=7
  In8 : Inport  Port=8
  In9 : Inport  Port=9
  In10 : Inport  Port=10
  In11 : Inport  Port=11
  In12 : Inport  Port=12
  In13 : Inport  Port=13
  In14 : Inport  Port=14
  In15 : Inport  Port=15
  In16 : Inport  Port=16
  In17 : Inport  Port=17
  In18 : Inport  Port=18
  In19 : Inport  Port=19
  In20 : Inport  Port=20
  Add : Sum  OutDataType=fixdt(1, 16)  OutScaling=2^-10
  Add1 : Sum  Inputs=+-  OutDataType=fixdt(1, 16)  OutScaling=2^-10
  Gain : Gain  Gain=K/N  ParameterDataType=fixdt(1, 16)  ParameterScaling=2^0  OutDataType=fixdt(1, 16)  OutScaling=2^0
  Integrator : Integrator  InitialConditionSource=external
  Mux : Mux  Inputs=20
  Scope : Scope
  Scope1 : Scope
  Sum of Elements : Sum  Inputs=+  OutDataType=fixdt(1, 16)  OutScaling=2^-10
  Threshold : Constant  Value=threshold  OutDataType=fixdt(1, 16)  OutScaling=2^0
  Trigonometric Function : Trigonometry
  angle speed : Constant  Value=omega  OutDataType=fixdt(1, 16)  OutScaling=2^0
  flash : Stateflow chart
  rho0 : Constant  Value=rho0+rand(1)*var  OutDataType=fixdt(1, 16)  OutScaling=2^0
  Out1 : Outport  OutDataType=fixdt(1, 16)  OutScaling=2^0
  wires:
  In20/1 -> Mux/20
  In19/1 -> Mux/19
  In18/1 -> Mux/18
  In17/1 -> Mux/17
  In16/1 -> Mux/16
  In15/1 -> Mux/15
  In14/1 -> Mux/14
  In13/1 -> Mux/13
  In12/1 -> Mux/12
  In11/1 -> Mux/11
  In10/1 -> Mux/10
  In9/1 -> Mux/9
  In8/1 -> Mux/8
  In7/1 -> Mux/7
  In6/1 -> Mux/6
  In5/1 -> Mux/5
  In4/1 -> Mux/4
  In3/1 -> Mux/3
  In2/1 -> Mux/2
  rho0/1 -> Integrator/2
  Threshold/1 -> flash/2(t)
  Sum of Elements/1 -> Gain/1
  Trigonometric Function/1 -> Sum of Elements/1
  Add/1 -> Scope1/1, flash/1(u), Integrator/1  "drho/dt"
  Gain/1 -> Add/2
  angle speed/1 -> Add/1
  Add1/1 -> Trigonometric Function/1
  Integrator/1 -> Scope/1, Out1/1, Add1/2  "rho_i"
  Mux/1 -> Add1/1
  In1/1 -> Mux/1

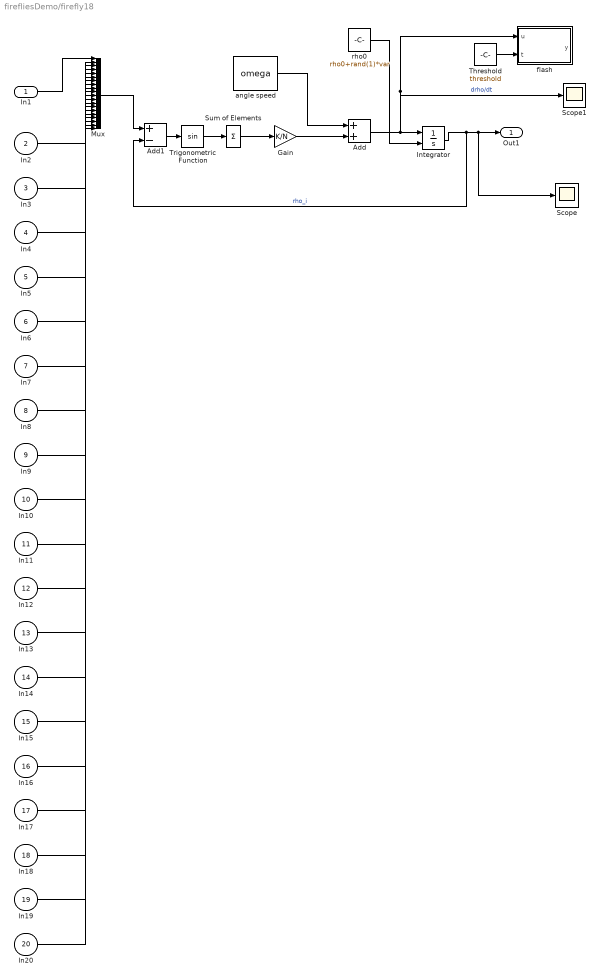
== system firefliesDemo/firefly18 ==
  In1 : Inport  OutDataType=fixdt(1, 16)  OutScaling=2^0
  In2 : Inport  Port=2
  In3 : Inport  Port=3
  In4 : Inport  Port=4
  In5 : Inport  Port=5
  In6 : Inport  Port=6
  In7 : Inport  Port=7
  In8 : Inport  Port=8
  In9 : Inport  Port=9
  In10 : Inport  Port=10
  In11 : Inport  Port=11
  In12 : Inport  Port=12
  In13 : Inport  Port=13
  In14 : Inport  Port=14
  In15 : Inport  Port=15
  In16 : Inport  Port=16
  In17 : Inport  Port=17
  In18 : Inport  Port=18
  In19 : Inport  Port=19
  In20 : Inport  Port=20
  Add : Sum  OutDataType=fixdt(1, 16)  OutScaling=2^-10
  Add1 : Sum  Inputs=+-  OutDataType=fixdt(1, 16)  OutScaling=2^-10
  Gain : Gain  Gain=K/N  ParameterDataType=fixdt(1, 16)  ParameterScaling=2^0  OutDataType=fixdt(1, 16)  OutScaling=2^0
  Integrator : Integrator  InitialConditionSource=external
  Mux : Mux  Inputs=20
  Scope : Scope
  Scope1 : Scope
  Sum of Elements : Sum  Inputs=+  OutDataType=fixdt(1, 16)  OutScaling=2^-10
  Threshold : Constant  Value=threshold  OutDataType=fixdt(1, 16)  OutScaling=2^0
  Trigonometric Function : Trigonometry
  angle speed : Constant  Value=omega  OutDataType=fixdt(1, 16)  OutScaling=2^0
  flash : Stateflow chart
  rho0 : Constant  Value=rho0+rand(1)*var  OutDataType=fixdt(1, 16)  OutScaling=2^0
  Out1 : Outport  OutDataType=fixdt(1, 16)  OutScaling=2^0
  wires:
  In20/1 -> Mux/20
  In19/1 -> Mux/19
  In18/1 -> Mux/18
  In17/1 -> Mux/17
  In16/1 -> Mux/16
  In15/1 -> Mux/15
  In14/1 -> Mux/14
  In13/1 -> Mux/13
  In12/1 -> Mux/12
  In11/1 -> Mux/11
  In10/1 -> Mux/10
  In9/1 -> Mux/9
  In8/1 -> Mux/8
  In7/1 -> Mux/7
  In6/1 -> Mux/6
  In5/1 -> Mux/5
  In4/1 -> Mux/4
  In3/1 -> Mux/3
  In2/1 -> Mux/2
  rho0/1 -> Integrator/2
  Threshold/1 -> flash/2(t)
  Sum of Elements/1 -> Gain/1
  Trigonometric Function/1 -> Sum of Elements/1
  Add/1 -> Scope1/1, flash/1(u), Integrator/1  "drho/dt"
  Gain/1 -> Add/2
  angle speed/1 -> Add/1
  Add1/1 -> Trigonometric Function/1
  Integrator/1 -> Scope/1, Out1/1, Add1/2  "rho_i"
  Mux/1 -> Add1/1
  In1/1 -> Mux/1

== system firefliesDemo/firefly19 ==
  In1 : Inport  OutDataType=fixdt(1, 16)  OutScaling=2^0
  In2 : Inport  Port=2
  In3 : Inport  Port=3
  In4 : Inport  Port=4
  In5 : Inport  Port=5
  In6 : Inport  Port=6
  In7 : Inport  Port=7
  In8 : Inport  Port=8
  In9 : Inport  Port=9
  In10 : Inport  Port=10
  In11 : Inport  Port=11
  In12 : Inport  Port=12
  In13 : Inport  Port=13
  In14 : Inport  Port=14
  In15 : Inport  Port=15
  In16 : Inport  Port=16
  In17 : Inport  Port=17
  In18 : Inport  Port=18
  In19 : Inport  Port=19
  In20 : Inport  Port=20
  Add : Sum  OutDataType=fixdt(1, 16)  OutScaling=2^-10
  Add1 : Sum  Inputs=+-  OutDataType=fixdt(1, 16)  OutScaling=2^-10
  Gain : Gain  Gain=K/N  ParameterDataType=fixdt(1, 16)  ParameterScaling=2^0  OutDataType=fixdt(1, 16)  OutScaling=2^0
  Integrator : Integrator  InitialConditionSource=external
  Mux : Mux  Inputs=20
  Scope : Scope
  Scope1 : Scope
  Sum of Elements : Sum  Inputs=+  OutDataType=fixdt(1, 16)  OutScaling=2^-10
  Threshold : Constant  Value=threshold  OutDataType=fixdt(1, 16)  OutScaling=2^0
  Trigonometric Function : Trigonometry
  angle speed : Constant  Value=omega  OutDataType=fixdt(1, 16)  OutScaling=2^0
  flash : Stateflow chart
  rho0 : Constant  Value=rho0+rand(1)*var  OutDataType=fixdt(1, 16)  OutScaling=2^0
  Out1 : Outport  OutDataType=fixdt(1, 16)  OutScaling=2^0
  wires:
  In20/1 -> Mux/20
  In19/1 -> Mux/19
  In18/1 -> Mux/18
  In17/1 -> Mux/17
  In16/1 -> Mux/16
  In15/1 -> Mux/15
  In14/1 -> Mux/14
  In13/1 -> Mux/13
  In12/1 -> Mux/12
  In11/1 -> Mux/11
  In10/1 -> Mux/10
  In9/1 -> Mux/9
  In8/1 -> Mux/8
  In7/1 -> Mux/7
  In6/1 -> Mux/6
  In5/1 -> Mux/5
  In4/1 -> Mux/4
  In3/1 -> Mux/3
  In2/1 -> Mux/2
  rho0/1 -> Integrator/2
  Threshold/1 -> flash/2(t)
  Sum of Elements/1 -> Gain/1
  Trigonometric Function/1 -> Sum of Elements/1
  Add/1 -> Scope1/1, flash/1(u), Integrator/1  "drho/dt"
  Gain/1 -> Add/2
  angle speed/1 -> Add/1
  Add1/1 -> Trigonometric Function/1
  Integrator/1 -> Scope/1, Out1/1, Add1/2  "rho_i"
  Mux/1 -> Add1/1
  In1/1 -> Mux/1

== system firefliesDemo/firefly2 ==
  In1 : Inport  OutDataType=fixdt(1, 16)  OutScaling=2^0
  In2 : Inport  Port=2
  In3 : Inport  Port=3
  In4 : Inport  Port=4
  In5 : Inport  Port=5
  In6 : Inport  Port=6
  In7 : Inport  Port=7
  In8 : Inport  Port=8
  In9 : Inport  Port=9
  In10 : Inport  Port=10
  In11 : Inport  Port=11
  In12 : Inport  Port=12
  In13 : Inport  Port=13
  In14 : Inport  Port=14
  In15 : Inport  Port=15
  In16 : Inport  Port=16
  In17 : Inport  Port=17
  In18 : Inport  Port=18
  In19 : Inport  Port=19
  In20 : Inport  Port=20
  Add : Sum  OutDataType=fixdt(1, 16)  OutScaling=2^-10
  Add1 : Sum  Inputs=+-  OutDataType=fixdt(1, 16)  OutScaling=2^-10
  Gain : Gain  Gain=K/N  ParameterDataType=fixdt(1, 16)  ParameterScaling=2^0  OutDataType=fixdt(1, 16)  OutScaling=2^0
  Integrator : Integrator  InitialConditionSource=external
  Mux : Mux  Inputs=20
  Scope : Scope
  Scope1 : Scope
  Sum of Elements : Sum  Inputs=+  OutDataType=fixdt(1, 16)  OutScaling=2^-10
  Threshold : Constant  Value=threshold  OutDataType=fixdt(1, 16)  OutScaling=2^0
  Trigonometric Function : Trigonometry
  angle speed : Constant  Value=omega  OutDataType=fixdt(1, 16)  OutScaling=2^0
  flash : Stateflow chart
  rho0 : Constant  Value=rho0+rand(1)*var  OutDataType=fixdt(1, 16)  OutScaling=2^0
  Out1 : Outport  OutDataType=fixdt(1, 16)  OutScaling=2^0
  wires:
  In20/1 -> Mux/20
  In19/1 -> Mux/19
  In18/1 -> Mux/18
  In17/1 -> Mux/17
  In16/1 -> Mux/16
  In15/1 -> Mux/15
  In14/1 -> Mux/14
  In13/1 -> Mux/13
  In12/1 -> Mux/12
  In11/1 -> Mux/11
  In10/1 -> Mux/10
  In9/1 -> Mux/9
  In8/1 -> Mux/8
  In7/1 -> Mux/7
  In6/1 -> Mux/6
  In5/1 -> Mux/5
  In4/1 -> Mux/4
  In3/1 -> Mux/3
  In2/1 -> Mux/2
  rho0/1 -> Integrator/2
  Threshold/1 -> flash/2(t)
  Sum of Elements/1 -> Gain/1
  Trigonometric Function/1 -> Sum of Elements/1
  Add/1 -> Scope1/1, flash/1(u), Integrator/1  "drho/dt"
  Gain/1 -> Add/2
  angle speed/1 -> Add/1
  Add1/1 -> Trigonometric Function/1
  Integrator/1 -> Scope/1, Out1/1, Add1/2  "rho_i"
  Mux/1 -> Add1/1
  In1/1 -> Mux/1

== system firefliesDemo/firefly3 ==
  In1 : Inport  OutDataType=fixdt(1, 16)  OutScaling=2^0
  In2 : Inport  Port=2
  In3 : Inport  Port=3
  In4 : Inport  Port=4
  In5 : Inport  Port=5
  In6 : Inport  Port=6
  In7 : Inport  Port=7
  In8 : Inport  Port=8
  In9 : Inport  Port=9
  In10 : Inport  Port=10
  In11 : Inport  Port=11
  In12 : Inport  Port=12
  In13 : Inport  Port=13
  In14 : Inport  Port=14
  In15 : Inport  Port=15
  In16 : Inport  Port=16
  In17 : Inport  Port=17
  In18 : Inport  Port=18
  In19 : Inport  Port=19
  In20 : Inport  Port=20
  Add : Sum  OutDataType=fixdt(1, 16)  OutScaling=2^-10
  Add1 : Sum  Inputs=+-  OutDataType=fixdt(1, 16)  OutScaling=2^-10
  Gain : Gain  Gain=K/N  ParameterDataType=fixdt(1, 16)  ParameterScaling=2^0  OutDataType=fixdt(1, 16)  OutScaling=2^0
  Integrator : Integrator  InitialConditionSource=external
  Mux : Mux  Inputs=20
  Scope : Scope
  Scope1 : Scope
  Sum of Elements : Sum  Inputs=+  OutDataType=fixdt(1, 16)  OutScaling=2^-10
  Threshold : Constant  Value=threshold  OutDataType=fixdt(1, 16)  OutScaling=2^0
  Trigonometric Function : Trigonometry
  angle speed : Constant  Value=omega  OutDataType=fixdt(1, 16)  OutScaling=2^0
  flash : Stateflow chart
  rho0 : Constant  Value=rho0+rand(1)*var  OutDataType=fixdt(1, 16)  OutScaling=2^0
  Out1 : Outport  OutDataType=fixdt(1, 16)  OutScaling=2^0
  wires:
  In20/1 -> Mux/20
  In19/1 -> Mux/19
  In18/1 -> Mux/18
  In17/1 -> Mux/17
  In16/1 -> Mux/16
  In15/1 -> Mux/15
  In14/1 -> Mux/14
  In13/1 -> Mux/13
  In12/1 -> Mux/12
  In11/1 -> Mux/11
  In10/1 -> Mux/10
  In9/1 -> Mux/9
  In8/1 -> Mux/8
  In7/1 -> Mux/7
  In6/1 -> Mux/6
  In5/1 -> Mux/5
  In4/1 -> Mux/4
  In3/1 -> Mux/3
  In2/1 -> Mux/2
  rho0/1 -> Integrator/2
  Threshold/1 -> flash/2(t)
  Sum of Elements/1 -> Gain/1
  Trigonometric Function/1 -> Sum of Elements/1
  Add/1 -> Scope1/1, flash/1(u), Integrator/1  "drho/dt"
  Gain/1 -> Add/2
  angle speed/1 -> Add/1
  Add1/1 -> Trigonometric Function/1
  Integrator/1 -> Scope/1, Out1/1, Add1/2  "rho_i"
  Mux/1 -> Add1/1
  In1/1 -> Mux/1

== system firefliesDemo/firefly4 ==
  In1 : Inport  OutDataType=fixdt(1, 16)  OutScaling=2^0
  In2 : Inport  Port=2
  In3 : Inport  Port=3
  In4 : Inport  Port=4
  In5 : Inport  Port=5
  In6 : Inport  Port=6
  In7 : Inport  Port=7
  In8 : Inport  Port=8
  In9 : Inport  Port=9
  In10 : Inport  Port=10
  In11 : Inport  Port=11
  In12 : Inport  Port=12
  In13 : Inport  Port=13
  In14 : Inport  Port=14
  In15 : Inport  Port=15
  In16 : Inport  Port=16
  In17 : Inport  Port=17
  In18 : Inport  Port=18
  In19 : Inport  Port=19
  In20 : Inport  Port=20
  Add : Sum  OutDataType=fixdt(1, 16)  OutScaling=2^-10
  Add1 : Sum  Inputs=+-  OutDataType=fixdt(1, 16)  OutScaling=2^-10
  Gain : Gain  Gain=K/N  ParameterDataType=fixdt(1, 16)  ParameterScaling=2^0  OutDataType=fixdt(1, 16)  OutScaling=2^0
  Integrator : Integrator  InitialConditionSource=external
  Mux : Mux  Inputs=20
  Scope : Scope
  Scope1 : Scope
  Sum of Elements : Sum  Inputs=+  OutDataType=fixdt(1, 16)  OutScaling=2^-10
  Threshold : Constant  Value=threshold  OutDataType=fixdt(1, 16)  OutScaling=2^0
  Trigonometric Function : Trigonometry
  angle speed : Constant  Value=omega  OutDataType=fixdt(1, 16)  OutScaling=2^0
  flash : Stateflow chart
  rho0 : Constant  Value=rho0+rand(1)*var  OutDataType=fixdt(1, 16)  OutScaling=2^0
  Out1 : Outport  OutDataType=fixdt(1, 16)  OutScaling=2^0
  wires:
  In20/1 -> Mux/20
  In19/1 -> Mux/19
  In18/1 -> Mux/18
  In17/1 -> Mux/17
  In16/1 -> Mux/16
  In15/1 -> Mux/15
  In14/1 -> Mux/14
  In13/1 -> Mux/13
  In12/1 -> Mux/12
  In11/1 -> Mux/11
  In10/1 -> Mux/10
  In9/1 -> Mux/9
  In8/1 -> Mux/8
  In7/1 -> Mux/7
  In6/1 -> Mux/6
  In5/1 -> Mux/5
  In4/1 -> Mux/4
  In3/1 -> Mux/3
  In2/1 -> Mux/2
  rho0/1 -> Integrator/2
  Threshold/1 -> flash/2(t)
  Sum of Elements/1 -> Gain/1
  Trigonometric Function/1 -> Sum of Elements/1
  Add/1 -> Scope1/1, flash/1(u), Integrator/1  "drho/dt"
  Gain/1 -> Add/2
  angle speed/1 -> Add/1
  Add1/1 -> Trigonometric Function/1
  Integrator/1 -> Scope/1, Out1/1, Add1/2  "rho_i"
  Mux/1 -> Add1/1
  In1/1 -> Mux/1

== system firefliesDemo/firefly5 ==
  In1 : Inport  OutDataType=fixdt(1, 16)  OutScaling=2^0
  In2 : Inport  Port=2
  In3 : Inport  Port=3
  In4 : Inport  Port=4
  In5 : Inport  Port=5
  In6 : Inport  Port=6
  In7 : Inport  Port=7
  In8 : Inport  Port=8
  In9 : Inport  Port=9
  In10 : Inport  Port=10
  In11 : Inport  Port=11
  In12 : Inport  Port=12
  In13 : Inport  Port=13
  In14 : Inport  Port=14
  In15 : Inport  Port=15
  In16 : Inport  Port=16
  In17 : Inport  Port=17
  In18 : Inport  Port=18
  In19 : Inport  Port=19
  In20 : Inport  Port=20
  Add : Sum  OutDataType=fixdt(1, 16)  OutScaling=2^-10
  Add1 : Sum  Inputs=+-  OutDataType=fixdt(1, 16)  OutScaling=2^-10
  Gain : Gain  Gain=K/N  ParameterDataType=fixdt(1, 16)  ParameterScaling=2^0  OutDataType=fixdt(1, 16)  OutScaling=2^0
  Integrator : Integrator  InitialConditionSource=external
  Mux : Mux  Inputs=20
  Scope : Scope
  Scope1 : Scope
  Sum of Elements : Sum  Inputs=+  OutDataType=fixdt(1, 16)  OutScaling=2^-10
  Threshold : Constant  Value=threshold  OutDataType=fixdt(1, 16)  OutScaling=2^0
  Trigonometric Function : Trigonometry
  angle speed : Constant  Value=omega  OutDataType=fixdt(1, 16)  OutScaling=2^0
  flash : Stateflow chart
  rho0 : Constant  Value=rho0+rand(1)*var  OutDataType=fixdt(1, 16)  OutScaling=2^0
  Out1 : Outport  OutDataType=fixdt(1, 16)  OutScaling=2^0
  wires:
  In20/1 -> Mux/20
  In19/1 -> Mux/19
  In18/1 -> Mux/18
  In17/1 -> Mux/17
  In16/1 -> Mux/16
  In15/1 -> Mux/15
  In14/1 -> Mux/14
  In13/1 -> Mux/13
  In12/1 -> Mux/12
  In11/1 -> Mux/11
  In10/1 -> Mux/10
  In9/1 -> Mux/9
  In8/1 -> Mux/8
  In7/1 -> Mux/7
  In6/1 -> Mux/6
  In5/1 -> Mux/5
  In4/1 -> Mux/4
  In3/1 -> Mux/3
  In2/1 -> Mux/2
  rho0/1 -> Integrator/2
  Threshold/1 -> flash/2(t)
  Sum of Elements/1 -> Gain/1
  Trigonometric Function/1 -> Sum of Elements/1
  Add/1 -> Scope1/1, flash/1(u), Integrator/1  "drho/dt"
  Gain/1 -> Add/2
  angle speed/1 -> Add/1
  Add1/1 -> Trigonometric Function/1
  Integrator/1 -> Scope/1, Out1/1, Add1/2  "rho_i"
  Mux/1 -> Add1/1
  In1/1 -> Mux/1

== system firefliesDemo/firefly6 ==
  In1 : Inport  OutDataType=fixdt(1, 16)  OutScaling=2^0
  In2 : Inport  Port=2
  In3 : Inport  Port=3
  In4 : Inport  Port=4
  In5 : Inport  Port=5
  In6 : Inport  Port=6
  In7 : Inport  Port=7
  In8 : Inport  Port=8
  In9 : Inport  Port=9
  In10 : Inport  Port=10
  In11 : Inport  Port=11
  In12 : Inport  Port=12
  In13 : Inport  Port=13
  In14 : Inport  Port=14
  In15 : Inport  Port=15
  In16 : Inport  Port=16
  In17 : Inport  Port=17
  In18 : Inport  Port=18
  In19 : Inport  Port=19
  In20 : Inport  Port=20
  Add : Sum  OutDataType=fixdt(1, 16)  OutScaling=2^-10
  Add1 : Sum  Inputs=+-  OutDataType=fixdt(1, 16)  OutScaling=2^-10
  Gain : Gain  Gain=K/N  ParameterDataType=fixdt(1, 16)  ParameterScaling=2^0  OutDataType=fixdt(1, 16)  OutScaling=2^0
  Integrator : Integrator  InitialConditionSource=external
  Mux : Mux  Inputs=20
  Scope : Scope
  Scope1 : Scope
  Sum of Elements : Sum  Inputs=+  OutDataType=fixdt(1, 16)  OutScaling=2^-10
  Threshold : Constant  Value=threshold  OutDataType=fixdt(1, 16)  OutScaling=2^0
  Trigonometric Function : Trigonometry
  angle speed : Constant  Value=omega  OutDataType=fixdt(1, 16)  OutScaling=2^0
  flash : Stateflow chart
  rho0 : Constant  Value=rho0+rand(1)*var  OutDataType=fixdt(1, 16)  OutScaling=2^0
  Out1 : Outport  OutDataType=fixdt(1, 16)  OutScaling=2^0
  wires:
  In20/1 -> Mux/20
  In19/1 -> Mux/19
  In18/1 -> Mux/18
  In17/1 -> Mux/17
  In16/1 -> Mux/16
  In15/1 -> Mux/15
  In14/1 -> Mux/14
  In13/1 -> Mux/13
  In12/1 -> Mux/12
  In11/1 -> Mux/11
  In10/1 -> Mux/10
  In9/1 -> Mux/9
  In8/1 -> Mux/8
  In7/1 -> Mux/7
  In6/1 -> Mux/6
  In5/1 -> Mux/5
  In4/1 -> Mux/4
  In3/1 -> Mux/3
  In2/1 -> Mux/2
  rho0/1 -> Integrator/2
  Threshold/1 -> flash/2(t)
  Sum of Elements/1 -> Gain/1
  Trigonometric Function/1 -> Sum of Elements/1
  Add/1 -> Scope1/1, flash/1(u), Integrator/1  "drho/dt"
  Gain/1 -> Add/2
  angle speed/1 -> Add/1
  Add1/1 -> Trigonometric Function/1
  Integrator/1 -> Scope/1, Out1/1, Add1/2  "rho_i"
  Mux/1 -> Add1/1
  In1/1 -> Mux/1

== system firefliesDemo/firefly7 ==
  In1 : Inport  OutDataType=fixdt(1, 16)  OutScaling=2^0
  In2 : Inport  Port=2
  In3 : Inport  Port=3
  In4 : Inport  Port=4
  In5 : Inport  Port=5
  In6 : Inport  Port=6
  In7 : Inport  Port=7
  In8 : Inport  Port=8
  In9 : Inport  Port=9
  In10 : Inport  Port=10
  In11 : Inport  Port=11
  In12 : Inport  Port=12
  In13 : Inport  Port=13
  In14 : Inport  Port=14
  In15 : Inport  Port=15
  In16 : Inport  Port=16
  In17 : Inport  Port=17
  In18 : Inport  Port=18
  In19 : Inport  Port=19
  In20 : Inport  Port=20
  Add : Sum  OutDataType=fixdt(1, 16)  OutScaling=2^-10
  Add1 : Sum  Inputs=+-  OutDataType=fixdt(1, 16)  OutScaling=2^-10
  Gain : Gain  Gain=K/N  ParameterDataType=fixdt(1, 16)  ParameterScaling=2^0  OutDataType=fixdt(1, 16)  OutScaling=2^0
  Integrator : Integrator  InitialConditionSource=external
  Mux : Mux  Inputs=20
  Scope : Scope
  Scope1 : Scope
  Sum of Elements : Sum  Inputs=+  OutDataType=fixdt(1, 16)  OutScaling=2^-10
  Threshold : Constant  Value=threshold  OutDataType=fixdt(1, 16)  OutScaling=2^0
  Trigonometric Function : Trigonometry
  angle speed : Constant  Value=omega  OutDataType=fixdt(1, 16)  OutScaling=2^0
  flash : Stateflow chart
  rho0 : Constant  Value=rho0+rand(1)*var  OutDataType=fixdt(1, 16)  OutScaling=2^0
  Out1 : Outport  OutDataType=fixdt(1, 16)  OutScaling=2^0
  wires:
  In20/1 -> Mux/20
  In19/1 -> Mux/19
  In18/1 -> Mux/18
  In17/1 -> Mux/17
  In16/1 -> Mux/16
  In15/1 -> Mux/15
  In14/1 -> Mux/14
  In13/1 -> Mux/13
  In12/1 -> Mux/12
  In11/1 -> Mux/11
  In10/1 -> Mux/10
  In9/1 -> Mux/9
  In8/1 -> Mux/8
  In7/1 -> Mux/7
  In6/1 -> Mux/6
  In5/1 -> Mux/5
  In4/1 -> Mux/4
  In3/1 -> Mux/3
  In2/1 -> Mux/2
  rho0/1 -> Integrator/2
  Threshold/1 -> flash/2(t)
  Sum of Elements/1 -> Gain/1
  Trigonometric Function/1 -> Sum of Elements/1
  Add/1 -> Scope1/1, flash/1(u), Integrator/1  "drho/dt"
  Gain/1 -> Add/2
  angle speed/1 -> Add/1
  Add1/1 -> Trigonometric Function/1
  Integrator/1 -> Scope/1, Out1/1, Add1/2  "rho_i"
  Mux/1 -> Add1/1
  In1/1 -> Mux/1

== system firefliesDemo/firefly8 ==
  In1 : Inport  OutDataType=fixdt(1, 16)  OutScaling=2^0
  In2 : Inport  Port=2
  In3 : Inport  Port=3
  In4 : Inport  Port=4
  In5 : Inport  Port=5
  In6 : Inport  Port=6
  In7 : Inport  Port=7
  In8 : Inport  Port=8
  In9 : Inport  Port=9
  In10 : Inport  Port=10
  In11 : Inport  Port=11
  In12 : Inport  Port=12
  In13 : Inport  Port=13
  In14 : Inport  Port=14
  In15 : Inport  Port=15
  In16 : Inport  Port=16
  In17 : Inport  Port=17
  In18 : Inport  Port=18
  In19 : Inport  Port=19
  In20 : Inport  Port=20
  Add : Sum  OutDataType=fixdt(1, 16)  OutScaling=2^-10
  Add1 : Sum  Inputs=+-  OutDataType=fixdt(1, 16)  OutScaling=2^-10
  Gain : Gain  Gain=K/N  ParameterDataType=fixdt(1, 16)  ParameterScaling=2^0  OutDataType=fixdt(1, 16)  OutScaling=2^0
  Integrator : Integrator  InitialConditionSource=external
  Mux : Mux  Inputs=20
  Scope : Scope
  Scope1 : Scope
  Sum of Elements : Sum  Inputs=+  OutDataType=fixdt(1, 16)  OutScaling=2^-10
  Threshold : Constant  Value=threshold  OutDataType=fixdt(1, 16)  OutScaling=2^0
  Trigonometric Function : Trigonometry
  angle speed : Constant  Value=omega  OutDataType=fixdt(1, 16)  OutScaling=2^0
  flash : Stateflow chart
  rho0 : Constant  Value=rho0+rand(1)*var  OutDataType=fixdt(1, 16)  OutScaling=2^0
  Out1 : Outport  OutDataType=fixdt(1, 16)  OutScaling=2^0
  wires:
  In20/1 -> Mux/20
  In19/1 -> Mux/19
  In18/1 -> Mux/18
  In17/1 -> Mux/17
  In16/1 -> Mux/16
  In15/1 -> Mux/15
  In14/1 -> Mux/14
  In13/1 -> Mux/13
  In12/1 -> Mux/12
  In11/1 -> Mux/11
  In10/1 -> Mux/10
  In9/1 -> Mux/9
  In8/1 -> Mux/8
  In7/1 -> Mux/7
  In6/1 -> Mux/6
  In5/1 -> Mux/5
  In4/1 -> Mux/4
  In3/1 -> Mux/3
  In2/1 -> Mux/2
  rho0/1 -> Integrator/2
  Threshold/1 -> flash/2(t)
  Sum of Elements/1 -> Gain/1
  Trigonometric Function/1 -> Sum of Elements/1
  Add/1 -> Scope1/1, flash/1(u), Integrator/1  "drho/dt"
  Gain/1 -> Add/2
  angle speed/1 -> Add/1
  Add1/1 -> Trigonometric Function/1
  Integrator/1 -> Scope/1, Out1/1, Add1/2  "rho_i"
  Mux/1 -> Add1/1
  In1/1 -> Mux/1
